simulink model "FMmod01"  (R2023b)
settings: Solver=VariableStepAuto  StartTime=0.0  StopTime=10.0  RelTol=1e-3
undefined symbols (not defined in the file or in its folder): FMmod, moduladora_L, moduladora_R
settings Model: Creator=garaya  LastModifiedBy=garaya

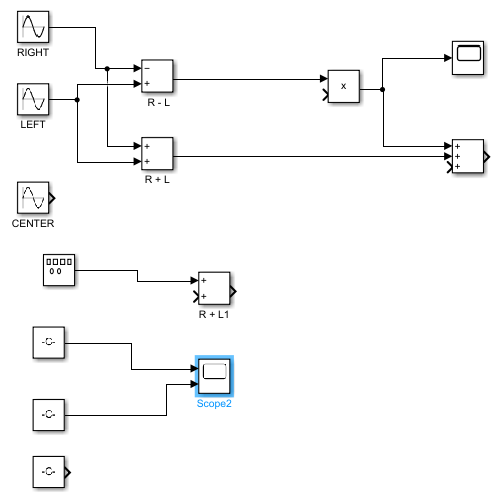
[thumbnail: Simulink's stored preview of the top-level diagram]
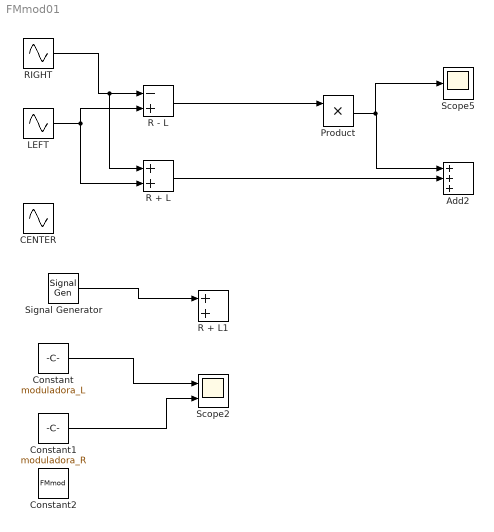
== system FMmod01 ==
  " R - L" : Sum  Inputs=-+
  Add2 : Sum  Inputs=+++
  CENTER : Sin  Frequency=33  SampleTime=0
  Constant : Constant  Value=moduladora_L
  Constant1 : Constant  Value=moduladora_R
  Constant2 : Constant  Value=FMmod
  LEFT : Sin  Frequency=200  SampleTime=0
  Product : Product
  R + L : Sum
  R + L1 : Sum
  RIGHT : Sin  Frequency=100  SampleTime=0
  Scope2 : Scope  NumInputPorts=2
  Scope5 : Scope
  Signal Generator : SignalGenerator  Frequency=2
  wires:
  LEFT/1 -> " R - L"/2, R + L/2
  RIGHT/1 -> R + L/1, " R - L"/1
  R + L/1 -> Add2/2
  " R - L"/1 -> Product/1
  Product/1 -> Scope5/1, Add2/1
  Signal Generator/1 -> R + L1/1
  Constant/1 -> Scope2/1
  Constant1/1 -> Scope2/2
